simulink model "Pod_trav_plant_mulecola"  (R2022b)
settings: Solver=VariableStepAuto  StartTime=0.0  StopTime=10.0  RelTol=1e-3
undefined symbols (not defined in the file): fix_constt, fric_gear_trav, JLrtg, JLrtt, JMrtg, JMrtt, Kktt, Kvtt
libraries: slctrlblks x1
settings Model: Creator=ohadformanair  LastModifiedBy=ohadformanair

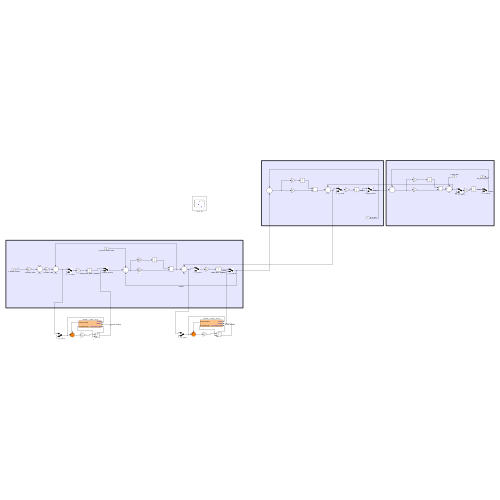
[thumbnail: Simulink's stored preview of the top-level diagram]
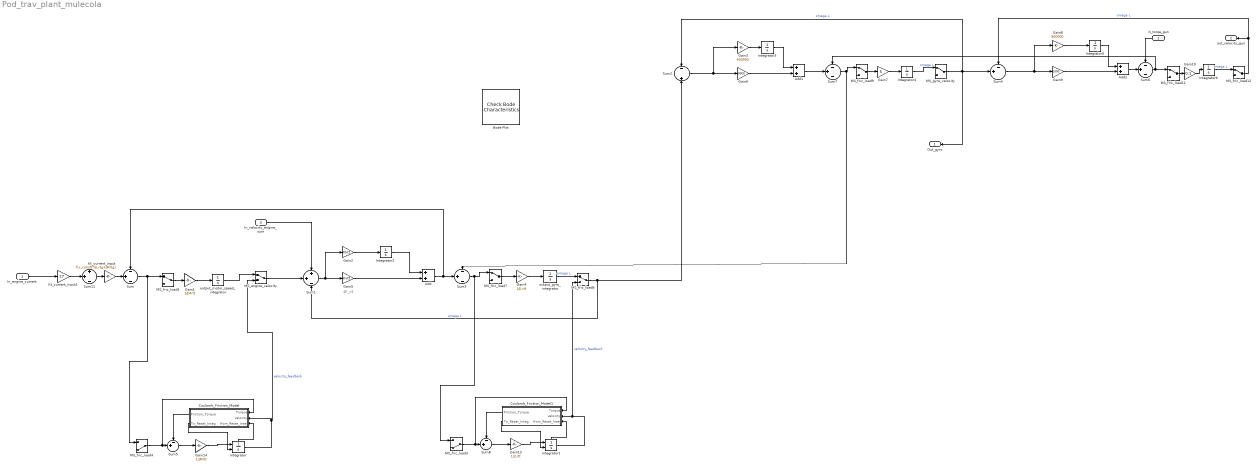
== system Pod_trav_plant_mulecola ==
  note: $K_v$
  In_engine_current : Inport
  in_torqe_gun : Inport  Port=2
  In_velocity_engine_sum : Inport  Port=3
  Add : Sum
  Add1 : Sum
  Add2 : Sum
  Bode Plot : slctrlblks/Model Verification/Check Bode  Characteristics  InstantiateOnLoad=on  SaveOperatingPoints=off  LinearizationIOs={'/In_engine_current', 1, 'in', 'off', '';'/MS_engine_velocity', 1, 'out', 'off', '';'/MS_gyro_velocity', 1, 'out', 'off', ''}  LinearizeAt=SnapshotTimes  SnapshotTimes=[0]  TriggerType=rising  SampleTime=auto  RateConversionMethod=zoh  PreWarpFreq=10  UseExactDelayModel=off  UseFullBlockNameLabels=off  UseBusSignalLabels=off  enabled=on  stopWhenAssertionFail=off  export=off  ViewDlgPos=[]  OpenViewOnLoad=off  LaunchViewOnOpen=off  FrequencyUnits=Hz  MagnitudeUnits=dB  PhaseUnits=deg  TimeUnits=seconds  EnableUpperBound=off  UpperBoundFrequencies=[]  UpperBoundMagnitudes=[]  EnableLowerBound=off  LowerBoundFrequencies=[]  LowerBoundMagnitudes=[]
      settings: LibrarySourceBlock=slctrlblks/Linear Analysis Plots/Bode Plot
  Coulomb_Friction_Model : Subsystem
  Coulomb_Friction_Model1 : Subsystem
  Gain1 : Gain  Gain=1/JMrtt
  Gain10 : Gain  Gain=0.1
  Gain13 : Gain  Gain=1/JLrtt
  Gain14 : Gain  Gain=1/JMrtt
  Gain2 : Gain  Gain=Kktt
  Gain3 : Gain  Gain=600000
  Gain4 : Gain  Gain=1/JLrtt
  Gain5 : Gain  Gain=Kvtt
  Gain6 : Gain  Gain=9000
  Gain7 : Gain  Gain=5
  Gain8 : Gain  Gain=800000
  Gain9 : Gain  Gain=1000
  Integrator : Integrator  ExternalReset=rising  ShowStatePort=on
  Integrator1 : Integrator  ExternalReset=rising  ShowStatePort=on
  Integrator{2..6} (5 alike) : Integrator
  Kt_current_input : Gain  Gain=fix_constt*(JLrtg+JMrtg)
  Kt_current_input1 : Gain  Gain=27
  MS_engine_velocity : ManualSwitch
  MS_fric_load{5,7..9,11..12} (6 alike) : ManualSwitch
  MS_fric_load3 : ManualSwitch  CurrentSetting=0
  MS_fric_load4 : ManualSwitch  CurrentSetting=0
  MS_gyro_velocity : ManualSwitch
  Sum{,3,6..7} (4 alike) : Sum  Inputs=-+-
  Sum1 : Sum  Inputs=++-
  Sum11 : Sum  Inputs=++-
  Sum2 : Sum  Inputs=-+
  Sum4 : Sum  Inputs=-+|
  Sum5 : Sum  Inputs=-+|  SaturateOnIntegerOverflow=on
  Sum8 : Sum  Inputs=-+|  SaturateOnIntegerOverflow=on
  output_gyro_integrator : Integrator
  output_motor_speed_integrator : Integrator
  Out_gyro : Outport
  out_velocity_gun : Outport  Port=2
  wires:
  Gain7/1 -> Integrator4/1
  Gain1/1 -> output_motor_speed_integrator/1
  Integrator5/1 -> Add2/1
  Integrator6/1 -> MS_fric_load12/1  "omega L"
  MS_gyro_velocity/1 -> Out_gyro/1, Sum2/1, Sum4/2  "omega L"
  MS_fric_load9/1 -> Gain7/1
  output_motor_speed_integrator/1 -> MS_engine_velocity/1
  Sum11/1 -> Kt_current_input/1
  Sum7/1 -> MS_fric_load9/1, Sum3/1
  Gain8/1 -> Integrator5/1
  Gain3/1 -> Integrator3/1
  Gain4/1 -> output_gyro_integrator/1
  Kt_current_input/1 -> Sum/2
  MS_fric_load8/1 -> Sum1/3, Sum2/2  "omega L"
  Gain6/1 -> Add1/2
  Integrator3/1 -> Add1/1
  Gain5/1 -> Add/2
  Integrator2/1 -> Add/1
  Integrator4/1 -> MS_gyro_velocity/1  "omega L"
  Gain2/1 -> Integrator2/1
  Sum6/1 -> Sum7/1, MS_fric_load11/1
  Sum/1 -> MS_fric_load4/1, MS_fric_load5/1
  MS_engine_velocity/1 -> Sum1/2
  Gain9/1 -> Add2/2
  Sum2/1 -> Gain6/1, Gain3/1
  Sum4/1 -> Gain9/1, Gain8/1
  MS_fric_load5/1 -> Gain1/1
  Gain10/1 -> Integrator6/1
  Sum1/1 -> Gain2/1, Gain5/1
  Add1/1 -> Sum7/2
  Add/1 -> Sum3/2, Sum/1
  output_gyro_integrator/1 -> MS_fric_load8/1  "omega L"
  Add2/1 -> Sum6/2
  MS_fric_load12/1 -> out_velocity_gun/1, Sum4/1  "omega L"
  MS_fric_load11/1 -> Gain10/1
  MS_fric_load7/1 -> Gain4/1
  In_engine_current/1 -> Kt_current_input1/1
  Kt_current_input1/1 -> Sum11/2
  in_torqe_gun/1 -> Sum6/1
  In_velocity_engine_sum/1 -> Sum1/1
  Gain14/1 -> Integrator/1
  Coulomb_Friction_Model/1(Friction_Torque) -> Sum5/1
  MS_fric_load4/1 -> Coulomb_Friction_Model/1(Torque), Sum5/2
  Integrator/1 -> MS_engine_velocity/2, Coulomb_Friction_Model/2(velocity)  "velocity_feedback"
  Coulomb_Friction_Model/2(To_Reset_Integ) -> Integrator/2
  Sum5/1 -> Gain14/1
  Integrator/State -> Coulomb_Friction_Model/3(from_Reset_Integ)
  Coulomb_Friction_Model1/2(To_Reset_Integ) -> Integrator1/2
  Integrator1/1 -> Coulomb_Friction_Model1/2(velocity), MS_fric_load8/2  "velocity_feedback"
  MS_fric_load3/1 -> Coulomb_Friction_Model1/1(Torque), Sum8/2
  Coulomb_Friction_Model1/1(Friction_Torque) -> Sum8/1
  Gain13/1 -> Integrator1/1
  Sum8/1 -> Gain13/1
  Sum3/1 -> MS_fric_load3/1, MS_fric_load7/1
  Integrator1/State -> Coulomb_Friction_Model1/3(from_Reset_Integ)

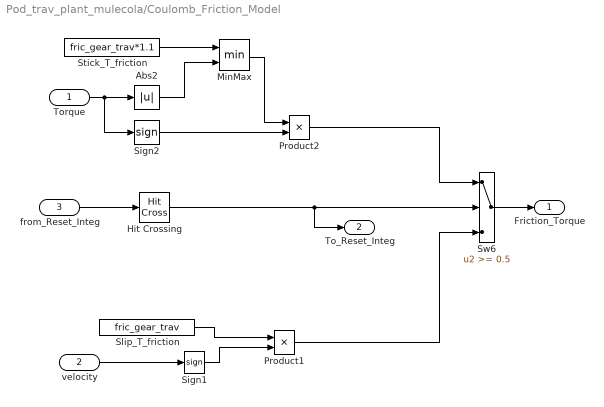
== system Pod_trav_plant_mulecola/Coulomb_Friction_Model ==
  Torque : Inport
  velocity : Inport  Port=2
  from_Reset_Integ : Inport  Port=3
  Abs2 : Abs  SaturateOnIntegerOverflow=off
  Hit Crossing : HitCross  ZeroCross=off
  MinMax : MinMax  Inputs=2
  Product1 : Product  RndMeth=Zero
  Product2 : Product  RndMeth=Zero
  Sign1 : Signum  ZeroCross=off
  Sign2 : Signum  ZeroCross=off
  Slip_T_friction : Constant  Value=fric_gear_trav
  Stick_T_friction : Constant  Value=fric_gear_trav*1.1
  Sw6 : Switch  Threshold=0.5
  Friction_Torque : Outport
  To_Reset_Integ : Outport  Port=2
  wires:
  Torque/1 -> Abs2/1, Sign2/1
  Sw6/1 -> Friction_Torque/1
  velocity/1 -> Sign1/1
  Sign1/1 -> Product1/2
  Product1/1 -> Sw6/3
  Hit Crossing/1 -> To_Reset_Integ/1, Sw6/2
  from_Reset_Integ/1 -> Hit Crossing/1
  Sign2/1 -> Product2/2
  Stick_T_friction/1 -> MinMax/1
  Abs2/1 -> MinMax/2
  MinMax/1 -> Product2/1
  Product2/1 -> Sw6/1
  Slip_T_friction/1 -> Product1/1

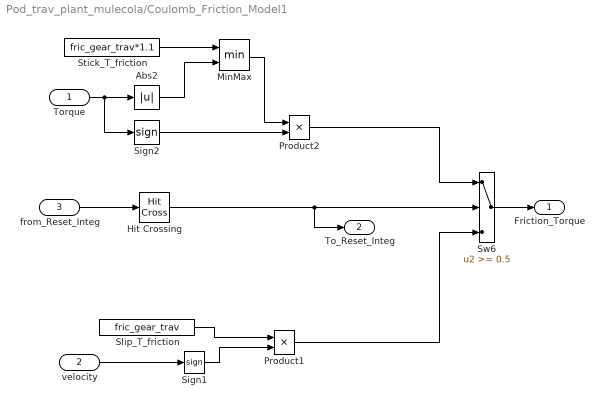
== system Pod_trav_plant_mulecola/Coulomb_Friction_Model1 ==
  Torque : Inport
  velocity : Inport  Port=2
  from_Reset_Integ : Inport  Port=3
  Abs2 : Abs  SaturateOnIntegerOverflow=off
  Hit Crossing : HitCross  ZeroCross=off
  MinMax : MinMax  Inputs=2
  Product1 : Product  RndMeth=Zero
  Product2 : Product  RndMeth=Zero
  Sign1 : Signum  ZeroCross=off
  Sign2 : Signum  ZeroCross=off
  Slip_T_friction : Constant  Value=fric_gear_trav
  Stick_T_friction : Constant  Value=fric_gear_trav*1.1
  Sw6 : Switch  Threshold=0.5
  Friction_Torque : Outport
  To_Reset_Integ : Outport  Port=2
  wires:
  Torque/1 -> Abs2/1, Sign2/1
  Sw6/1 -> Friction_Torque/1
  velocity/1 -> Sign1/1
  Sign1/1 -> Product1/2
  Product1/1 -> Sw6/3
  Hit Crossing/1 -> To_Reset_Integ/1, Sw6/2
  from_Reset_Integ/1 -> Hit Crossing/1
  Sign2/1 -> Product2/2
  Stick_T_friction/1 -> MinMax/1
  Abs2/1 -> MinMax/2
  MinMax/1 -> Product2/1
  Product2/1 -> Sw6/1
  Slip_T_friction/1 -> Product1/1
